simulink model "SynthFSE"  (R2019a)
settings: Solver=ode45  StartTime=0.0  StopTime=1780  RelTol=1e-3  EnableMultiTasking=on
undefined symbols (not defined in the file): j
libraries: xbsIndex_r4 x72, dspmlti4 x2, xbsCopyrightNotice_r4 x1
(part 1 of 2)
settings Model: Creator=alexc  LastModifiedBy=viswanad
settings DataIOCC: LimitDataPoints=on  SaveFormat=Array  SignalLoggingSaveFormat=ModelDataLogs  ReturnWorkspaceOutputs=off  SignalLoggingName=sigsOut
settings OptimizationCC: BlockReduction=off  BooleanDataType=off  ExpressionDepthLimit=2147483647  InitFltsAndDblsToZero=on  LifeSpan=inf
settings DebuggingCC: SaveWithParameterizedLinksMsg=none  UnderspecifiedInitializationDetection=Classic  MergeDetectMultiDrivingBlocksExec=none  SignalResolutionControl=TryResolveAllWithWarning  MultiTaskDSMMsg=warning  MultiTaskCondExecSysMsg=none  FcnCallInpInsideContextMsg=warning  StateNameClashWarn=warning  SFUnexpectedBacktrackingDiag=warning  SFNoUnconditionalDefaultTransitionDiag=warning  SFExecutionAtInitializationDiag=none  ArithmeticOperatorsInVariantConditions=warning
settings HardwareCC: ProdBitPerPointer=32  ProdBitPerSizeT=32  ProdBitPerPtrDiffT=32  ProdLargestAtomicFloat=None  ProdIntDivRoundTo=Undefined  ProdEndianess=Unspecified  ProdWordSize=32  ProdHWDeviceType=32-bit Generic  TargetUnknown=on
settings ModelReferenceCC: PropagateSignalLabelsOutOfModel=off
settings SFSimCC: SimUseLocalCustomCode=off
settings RTWCC: Description=Generic Real-Time Target  RTWUseLocalCustomCode=off
settings CodeAppCC: StateflowObjectComments=on
settings GRTTargetCC: TargetFcnLib=ansi_tfl_tmw.mat  TargetLangStandard=C89/C90 (ANSI)  GeneratePreprocessorConditionals=Disable all  CombineOutputUpdateFcns=off  GRTInterface=on
settings ConfigComp: CovMetricSettings=dw  CovHtmlReporting=on  CovSaveCumulativeToWorkspaceVar=on  CovSaveSingleToWorkspaceVar=on  CovExternalEMLEnable=off

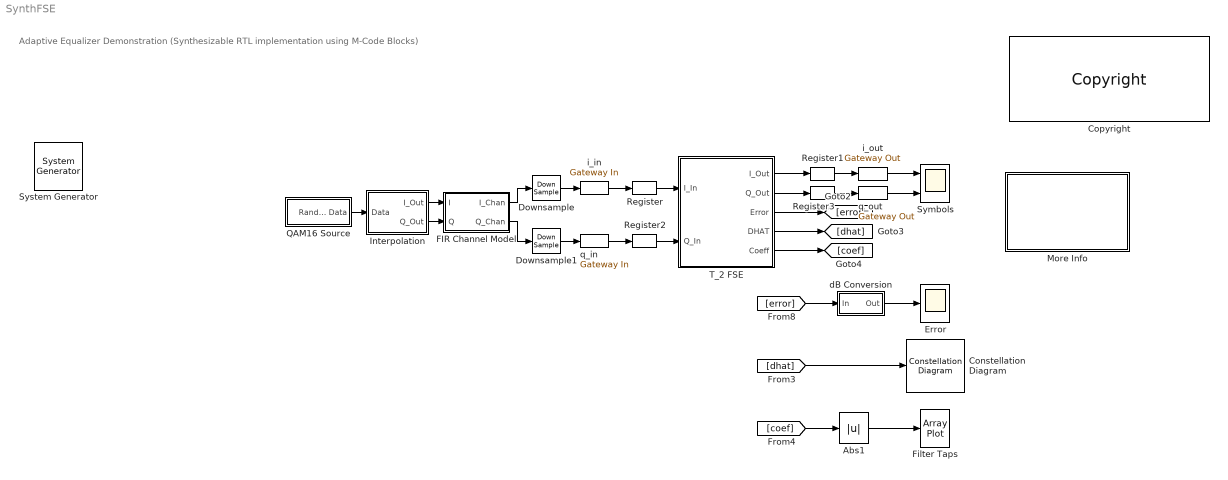
== system SynthFSE ==
  note: Adaptive Equalizer Demonstration
      | (Synthesizable RTL implementation using M-Code Blocks)
  " System Generator" : xbsIndex_r4/ System Generator  Tag=genX  xilinxfamily=kintex7  part=xc7k325t  speed=-3  package=fbg676  synthesis_tool=Vivado  clock_wrapper=Clock Enables  directory=./netlist  proj_type=Vivado  Synth_file=Vivado Synthesis Defaults  Impl_file=Vivado Implementation Defaults  testbench=off  simulink_period=1  sysclk_period=10  dcm_input_clock_period=10  incr_netlist=off  trim_vbits=Everywhere in SubSystem  dbl_ovrd=According to Block Masks  core_generation=According to Block Masks  run_coregen=off  deprecated_control=off  eval_field=0  block_type=sysgen
  Abs1 : Abs  SaturateOnIntegerOverflow=on
  Constellation Diagram : ConstellationDiagram
  Copyright : xbsCopyrightNotice_r4/Copyright  copyrighttext="Copyright (c) 2020  by  Xilinx, Inc. All rights reserved.<br><br>This file contains proprietary, confidential information of Xilinx, Inc., is distributed under license from Xilinx, Inc., and may be used, copied and/or disclosed only pursuant to the terms of a valid license agreement with Xilinx, Inc. Xilinx hereby grants you a license to use this file solely for design, simulation, implementation and creation of design files limited to Xilinx devices or technologies. Use with non-Xilinx devices or technologies is expressly prohibited and immediately terminates your license unless covered by a separate agreement.<br><br>Xilinx is providing this design, code, or information \"as-is\" solely for use in developing programs and solutions for Xilinx devices, with no obligation on the part of Xilinx to provide support. By providing this design, code, or information as one possible implementation of this feature, application or standard, Xilinx is making no representation that this implementation is free from any claims of infringement. You are responsible for obtaining any rights you may require for your implementation. Xilinx expressly disclaims any warranty whatsoever with respect to the adequacy of the implementation, including but not limited to any warranties or representations that this implementation is free from claims of infringement, implied warranties of merchantability or fitness for a particular purpose.<br><br>Xilinx products are not intended for use in life support appliances, devices, or systems. Use in such applications is expressly prohibited.<br><br>Any modifications that are made to the Source Code are done at the user's sole risk and will be unsupported.<br><br>This copyright and support notice must be retained as part of this text at all times. (c) Copyright 1995-2020 Xilinx, Inc. All rights reserved."  block_type=copyright
      settings: block_version=10.1.00
      settings: infoedit=|
      | Copyright(C) 2008 by  Xilinx, Inc. All rights reserved.<br>
      | <br>
      | This file contains proprietary, confidential information of Xilinx, Inc., is distributed under license
      | from Xilinx, Inc., and may be used, copied and/or disclosed only pursuant to the terms of a valid license
      | agreement with Xilinx, Inc. Xilinx hereby grants you a license to use this file solely for design,
      | simulation, implementation and creation of design files limited to Xilinx devices or technologies. Use
      | with non-Xilinx devices or technologies is expressly prohibited and immediately terminates your license
      | unless covered by a separate agreement.<br>
      | <br>
      | Xilinx is providing this design, code, or information "as-is" solely for use in developing programs and
      | solutions for Xilinx devices, with no obligation on the part of Xilinx to provide support. By providing
      | this design, code, or information as one possible implementation of this feature, application or standard,
      | Xilinx is making no representation that this implementation is free from any claims of infringement. You
      | are responsible for obtaining any rights you may require for your implementation. Xilinx expressly disclaims
      | any warranty whatsoever with respect to the adequacy of the implementation, including but not limited to any
      | warranties or representations that this implementation is free from claims of infringement, implied warranties
      | of merchantability or fitness for a particular purpose.<br>
      | <br>
      | Xilinx products are not intended for use in life support appliances, devices, or systems. Use in such
      | applications is expressly prohibited.<br>
      | <br>
      | Any modifications that are made to the Source Code are done at the user's sole risk and will be unsupported.<br>
      | <br>
      | This copyright and support notice must be retained as part of this text at all times.
      | (c) Copyright 1995-2008 Xilinx, Inc. All rights reserved.
  Downsample : DownSample  RateOptions=Allow multirate processing
  Downsample1 : DownSample  RateOptions=Allow multirate processing
  Error : Scope
  FIR Channel Model : Subsystem  mask{chan=[1+j*0.1 .2 j*0.2 0 0 0 0 0 0 0]}
      mask prompts: chan "Channel"
  Filter Taps : ArrayPlot
  Interpolation : Subsystem
  More Info : Subsystem
      mask Display: disp('Double click\n for\n more information.')
  QAM16 Source : Subsystem
  Register{,1..3} (4 alike) : xbsIndex_r4/Register  init=0  rst=off  en=off  dbl_ovrd=off  block_type=register
      Register settings: xl_area=[6 12 0 0 0 0 0]  block_version=VER_STRING_GOES_HERE
      Register1 settings: xl_area=[5 10 0 0 0 0 0]  block_version=VER_STRING_GOES_HERE
      Register2 settings: xl_area=[6 12 0 0 0 0 0]  block_version=VER_STRING_GOES_HERE
      Register3 settings: xl_area=[5 10 0 0 0 0 0]  block_version=VER_STRING_GOES_HERE
  Symbols : Scope  NumInputPorts=2
  T_2 FSE : Subsystem  mask{mu=.005}
  dB Conversion : Subsystem
  i_in : xbsIndex_r4/Gateway In  gui_display_data_type=Fixed-point  arith_type="Signed  (2's comp)"  n_bits=12  bin_pt=10  preci_type=Single  exp_width=8  frac_width=24  rows=1  columns=1  quantization="Round  (unbiased: +/- Inf)"  overflow=Saturate  period=2  UseAsADC=off  ADCChannel='1'  interface=None  automatic_assignment=on  address_offset=hex2dec('00')  intf_name=''  intf_description=''  default_value=0  timing_constraint=None  locs_specified=off  LOCs={}  io_standard={}  inherit_from_input=off  hdl_port=on  dbl_ovrd=off  block_type=gatewayin
      settings: infoedit="Gateway in block.  Converts inputs of type Simulink integer, double and fixed point to  Xilinx fixed point type.<P><P>Hardware notes:  In hardware these blocks become top level input ports."  xl_area=[0 0 0 0 12 0 0]  block_version=VER_STRING_GOES_HERE
  i_out : xbsIndex_r4/Gateway Out  inherit_from_input=off  hdl_port=on  rows=1  columns=1  UseAsDAC=off  DACChannel='1'  interface=None  automatic_assignment=on  address_offset=hex2dec('00')  intf_name=''  intf_description=''  timing_constraint="Data Rate;  Set 'FAST' Attribute"  locs_specified=off  LOCs={}  io_standard={}  block_type=gatewayout
      settings: infoedit="Gateway out block.  Converts Xilinx fixed point inputs into ouputs of type Simulink integer, double, or fixed point.<P><P>Hardware notes:  In hardware these blocks become top level output ports or are discarded, depending on how they are configured."  xl_area=[0 0 0 0 10 0 0]  block_version=VER_STRING_GOES_HERE
  q_in : xbsIndex_r4/Gateway In  gui_display_data_type=Fixed-point  arith_type="Signed  (2's comp)"  n_bits=12  bin_pt=10  preci_type=Single  exp_width=8  frac_width=24  rows=1  columns=1  quantization="Round  (unbiased: +/- Inf)"  overflow=Saturate  period=2  UseAsADC=off  ADCChannel='1'  interface=None  automatic_assignment=on  address_offset=hex2dec('00')  intf_name=''  intf_description=''  default_value=0  timing_constraint=None  locs_specified=off  LOCs={}  io_standard={}  inherit_from_input=off  hdl_port=on  dbl_ovrd=off  block_type=gatewayin
      settings: infoedit="Gateway in block.  Converts inputs of type Simulink integer, double and fixed point to  Xilinx fixed point type.<P><P>Hardware notes:  In hardware these blocks become top level input ports."  xl_area=[0 0 0 0 12 0 0]  block_version=VER_STRING_GOES_HERE
  q_out : xbsIndex_r4/Gateway Out  inherit_from_input=off  hdl_port=on  rows=1  columns=1  UseAsDAC=off  DACChannel='1'  interface=None  automatic_assignment=on  address_offset=hex2dec('00')  intf_name=''  intf_description=''  timing_constraint="Data Rate;  Set 'FAST' Attribute"  locs_specified=off  LOCs={}  io_standard={}  block_type=gatewayout
      settings: infoedit="Gateway out block.  Converts Xilinx fixed point inputs into ouputs of type Simulink integer, double, or fixed point.<P><P>Hardware notes:  In hardware these blocks become top level output ports or are discarded, depending on how they are configured."  xl_area=[0 0 0 0 10 0 0]  block_version=VER_STRING_GOES_HERE
  wires:
  QAM16 Source/1(" Random Data") -> Interpolation/1(Data)
  Interpolation/2(Q_Out) -> FIR Channel Model/2(Q)
  T_2 FSE/3(Error) -> [error]
  Downsample1/1 -> q_in/1
  Downsample/1 -> i_in/1
  Interpolation/1(I_Out) -> FIR Channel Model/1(I)
  T_2 FSE/2(Q_Out) -> Register3/1
  T_2 FSE/1(I_Out) -> Register1/1
  FIR Channel Model/1(I_Chan) -> Downsample/1
  FIR Channel Model/2(Q_Chan) -> Downsample1/1
  T_2 FSE/5(Coeff) -> [coef]
  i_in/1 -> Register/1
  Abs1/1 -> Filter Taps/1
  T_2 FSE/4(DHAT) -> [dhat]
  dB Conversion/1(Out) -> Error/1
  Register2/1 -> T_2 FSE/2(Q_In)
  Register1/1 -> i_out/1
  Register3/1 -> q_out/1
  q_in/1 -> Register2/1
  Register/1 -> T_2 FSE/1(I_In)
  [coef] -> Abs1/1
  [dhat] -> Constellation Diagram/1
  [error] -> dB Conversion/1(In)
  i_out/1 -> Symbols/1
  q_out/1 -> Symbols/2

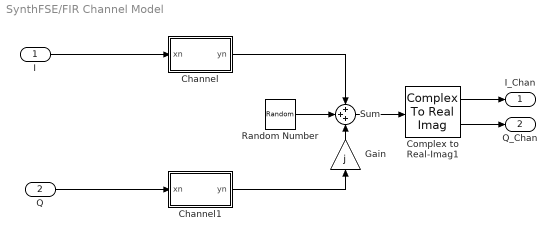
== system SynthFSE/FIR Channel Model ==
  I : Inport
  Q : Inport  Port=2
  Channel : Subsystem
  Channel1 : Subsystem
  Complex to Real-Imag1 : ComplexToRealImag
  Gain : Gain  Gain=j  SaturateOnIntegerOverflow=on  OutDataTypeStr=Inherit: Same as input  ParamDataTypeStr=Inherit: Same as input
  Random Number : RandomNumber  Variance=.01  SampleTime=100000
  Sum : Sum  Inputs=+++  SaturateOnIntegerOverflow=on  InputSameDT=on  OutDataTypeStr=Inherit: Same as first input
  I_Chan : Outport
  Q_Chan : Outport  Port=2
  wires:
  Channel1/1(yn) -> Gain/1
  Channel/1(yn) -> Sum/1
  Q/1 -> Channel1/1(xn)
  I/1 -> Channel/1(xn)
  Random Number/1 -> Sum/2
  Gain/1 -> Sum/3
  Sum/1 -> Complex to Real-Imag1/1
  Complex to Real-Imag1/2 -> Q_Chan/1
  Complex to Real-Imag1/1 -> I_Chan/1

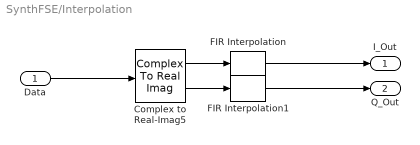
== system SynthFSE/Interpolation ==
  Data : Inport
  Complex to Real-Imag5 : ComplexToRealImag
  FIR Interpolation : dspmlti4/FIR Interpolation  FilterSource=Dialog parameters  h=sinc(-3:.25:3);  L=4  FilterObject=Hm_firinterp  framing=Allow multirate processing  outputBufInitCond=0  roundingMode=Floor  overflowMode=off  firstCoeffDataTypeStr=Inherit: Same word length as input  firstCoeffMin=[]  firstCoeffMax=[]  firstCoeffLastDataTypeStr=Inherit: Same word length as input  outputDataTypeStr=Inherit: Same as accumulator  outputMin=[]  outputMax=[]  outputLastDataTypeStr=Inherit: Same as accumulator
      settings: SourceProductName=DSP System Toolbox
  FIR Interpolation1 : dspmlti4/FIR Interpolation  FilterSource=Dialog parameters  h=sinc(-3:.25:3);  L=4  FilterObject=Hm_firinterp  framing=Allow multirate processing  outputBufInitCond=0  roundingMode=Floor  overflowMode=off  firstCoeffDataTypeStr=Inherit: Same word length as input  firstCoeffMin=[]  firstCoeffMax=[]  firstCoeffLastDataTypeStr=Inherit: Same word length as input  outputDataTypeStr=Inherit: Same as accumulator  outputMin=[]  outputMax=[]  outputLastDataTypeStr=Inherit: Same as accumulator
      settings: SourceProductName=DSP System Toolbox
  I_Out : Outport
  Q_Out : Outport  Port=2
  wires:
  Complex to Real-Imag5/2 -> FIR Interpolation1/1
  Complex to Real-Imag5/1 -> FIR Interpolation/1
  FIR Interpolation/1 -> I_Out/1
  Data/1 -> Complex to Real-Imag5/1
  FIR Interpolation1/1 -> Q_Out/1

== system SynthFSE/More Info ==
  note: This design shows a T/2 adaptive Fractionally Space Equalizer (FSE)
      | operating on a 16-QAM data source with noise and filtering introduced
      | in the channel model.  The two 4-tap FIR filters are based on an
      | SRL16E-based MAC implementation.
      |
      | The DHAT scope provides an X-Y plot of the I and Q filter outputs from
      | within the FSE.  As the simulation progresses, these symbols will
      | converge as the error is reduced.  The magnitude of the filter coefficients
      | is shown in a vector scope as well.  Increasing the simulation duration
      | will allow better visualization of the adaptive FSE effects on the filter output.
      |
      | For additional information on FSE:
      |
      | J.R. Treichler, I. Fijalkow, and C.R. Johnson, Jr.  "Fractionally Spaced
      | Equalizers"  IEEE Signal Processing Magazine, May 1996, pp. 65-81.
      |
      | Chris H. Dick, "Design and implementation of high-performance FPGA
      | signal processing datapaths for software-defined radios" VMEbus
      | Systems, August 2001.
  note: Adaptive FSE Demonstration Using a 16-QAM Source

== system SynthFSE/QAM16 Source ==
  QAM16 - I : Subsystem
  QAM16 -Q : Subsystem
  Real-Imag to Complex : RealImagToComplex
  " Random Data" : Outport
  wires:
  QAM16 - I/1(I) -> Real-Imag to Complex/1
  QAM16 -Q/1(Q) -> Real-Imag to Complex/2
  Real-Imag to Complex/1 -> " Random Data"/1

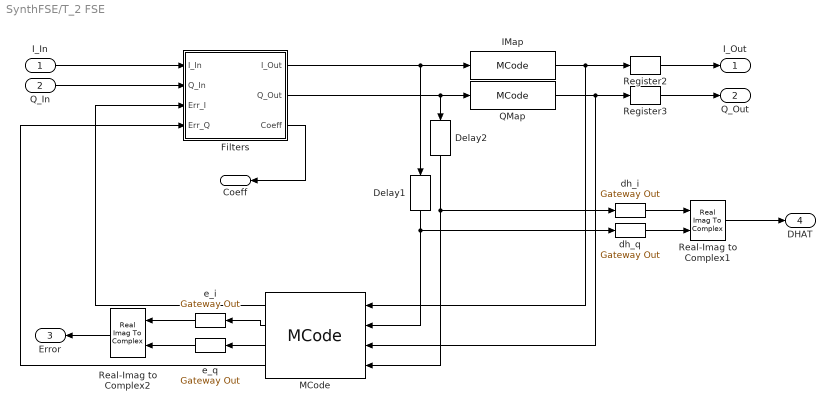
== system SynthFSE/T_2 FSE ==
  I_In : Inport
  Q_In : Inport  Port=2
  Delay1 : xbsIndex_r4/Delay  rst=off  infoeditControl=Selection of Reset will increase slice count due to use of real FFs and instead of SRLs  en=off  latency=2  reg_retiming=on  dbl_ovrd=off  block_type=delay
      settings: infoedit="Delay line having  configurable length.<P><P>Hardware notes: A delay line is a chain, each link of which is an SRL16 followed by a flip-flop. If register retiming is enabled, the delay line is a chain of flip-flops."  xl_area=[9 18 0 18 0 0 0]  block_version=VER_STRING_GOES_HERE
  Delay2 : xbsIndex_r4/Delay  rst=off  infoeditControl=Selection of Reset will increase slice count due to use of real FFs and instead of SRLs  en=off  latency=2  reg_retiming=on  dbl_ovrd=off  block_type=delay
      settings: infoedit="Delay line having  configurable length.<P><P>Hardware notes: A delay line is a chain, each link of which is an SRL16 followed by a flip-flop. If register retiming is enabled, the delay line is a chain of flip-flops."  xl_area=[9 18 0 18 0 0 0]  block_version=VER_STRING_GOES_HERE
  Filters : Subsystem
  IMap : xbsIndex_r4/MCode  mfname=QAM4map  explicit_period=off  period=1  enable_stdout=off  enable_debug=off  suppress_output=off  defparams={}  hide_port_list={}  dbl_ovrd=off  block_type=mcode
      settings: xl_area=[0, 0, 0, 0, 0, 0, 0]  block_version=8.1
  MCode : xbsIndex_r4/MCode  mfname=lmsErr  explicit_period=off  period=1  inputsTable={'boundInpExpr'=>['','','','','mu'],'inputs'=>['sym_i','filt_i','sym_q','filt_q','mu']}  outputsTable={'outputs'=>['mu_e_i','e_i','e_q','mu_e_q'],'suppressOut'=>['off','off','off','off']}  enable_stdout=off  enable_debug=off  suppress_output=1  defparams={'mu',mu}  hide_port_list={}  dbl_ovrd=off  block_type=mcode
      settings: block_version=8.2.EA1
  QMap : xbsIndex_r4/MCode  mfname=QAM4map  explicit_period=off  period=1  enable_stdout=off  enable_debug=off  suppress_output=off  defparams={}  hide_port_list={}  dbl_ovrd=off  block_type=mcode
      settings: xl_area=[0, 0, 0, 0, 0, 0, 0]  block_version=8.1
  Real-Imag to Complex1 : RealImagToComplex
  Real-Imag to Complex2 : RealImagToComplex
  Register2 : xbsIndex_r4/Register  init=0  rst=off  en=off  dbl_ovrd=off  block_type=register
      settings: xl_area=[5 10 0 0 0 0 0]  block_version=VER_STRING_GOES_HERE
  Register3 : xbsIndex_r4/Register  init=0  rst=off  en=off  dbl_ovrd=off  block_type=register
      settings: xl_area=[5 10 0 0 0 0 0]  block_version=VER_STRING_GOES_HERE
  dh_i : xbsIndex_r4/Gateway Out  inherit_from_input=off  hdl_port=off  rows=1  columns=1  UseAsDAC=off  DACChannel='1'  interface=None  automatic_assignment=on  address_offset=hex2dec('00')  intf_name=''  intf_description=''  timing_constraint=None  locs_specified=off  LOCs={}  io_standard={}  block_type=gatewayout
      settings: infoedit="Gateway out block.  Converts Xilinx fixed point inputs into ouputs of type Simulink integer, double, or fixed point.<P><P>Hardware notes:  In hardware these blocks become top level output ports or are discarded, depending on how they are configured."  xl_area=[0 0 0 0 0 0 0]  block_version=VER_STRING_GOES_HERE
  dh_q : xbsIndex_r4/Gateway Out  inherit_from_input=off  hdl_port=off  rows=1  columns=1  UseAsDAC=off  DACChannel='1'  interface=None  automatic_assignment=on  address_offset=hex2dec('00')  intf_name=''  intf_description=''  timing_constraint=None  locs_specified=off  LOCs={}  io_standard={}  block_type=gatewayout
      settings: infoedit="Gateway out block.  Converts Xilinx fixed point inputs into ouputs of type Simulink integer, double, or fixed point.<P><P>Hardware notes:  In hardware these blocks become top level output ports or are discarded, depending on how they are configured."  xl_area=[0 0 0 0 0 0 0]  block_version=VER_STRING_GOES_HERE
  e_i : xbsIndex_r4/Gateway Out  inherit_from_input=off  hdl_port=off  rows=1  columns=1  UseAsDAC=off  DACChannel='1'  interface=None  automatic_assignment=on  address_offset=hex2dec('00')  intf_name=''  intf_description=''  timing_constraint=None  locs_specified=off  LOCs={}  io_standard={}  block_type=gatewayout
      settings: infoedit="Gateway out block.  Converts Xilinx fixed point inputs into ouputs of type Simulink integer, double, or fixed point.<P><P>Hardware notes:  In hardware these blocks become top level output ports or are discarded, depending on how they are configured."  xl_area=[0 0 0 0 0 0 0]  block_version=VER_STRING_GOES_HERE
  e_q : xbsIndex_r4/Gateway Out  inherit_from_input=off  hdl_port=off  rows=1  columns=1  UseAsDAC=off  DACChannel='1'  interface=None  automatic_assignment=on  address_offset=hex2dec('00')  intf_name=''  intf_description=''  timing_constraint=None  locs_specified=off  LOCs={}  io_standard={}  block_type=gatewayout
      settings: infoedit="Gateway out block.  Converts Xilinx fixed point inputs into ouputs of type Simulink integer, double, or fixed point.<P><P>Hardware notes:  In hardware these blocks become top level output ports or are discarded, depending on how they are configured."  xl_area=[0 0 0 0 0 0 0]  block_version=VER_STRING_GOES_HERE
  I_Out : Outport
  Q_Out : Outport  Port=2
  Error : Outport  Port=3
  DHAT : Outport  Port=4
  Coeff : Outport  Port=5
  wires:
  Q_In/1 -> Filters/2(Q_In)
  Filters/1(I_Out) -> Delay1/1, IMap/1
  QMap/1 -> Register3/1, MCode/3
  IMap/1 -> Register2/1, MCode/1
  Filters/2(Q_Out) -> Delay2/1, QMap/1
  I_In/1 -> Filters/1(I_In)
  Delay1/1 -> dh_q/1, MCode/2
  Delay2/1 -> dh_i/1, MCode/4
  Real-Imag to Complex1/1 -> DHAT/1
  dh_i/1 -> Real-Imag to Complex1/1
  dh_q/1 -> Real-Imag to Complex1/2
  Filters/3(Coeff) -> Coeff/1
  Register2/1 -> I_Out/1
  Register3/1 -> Q_Out/1
  e_i/1 -> Real-Imag to Complex2/1
  e_q/1 -> Real-Imag to Complex2/2
  MCode/2 -> e_i/1
  MCode/3 -> e_q/1
  Real-Imag to Complex2/1 -> Error/1
  MCode/1 -> Filters/3(Err_I)
  MCode/4 -> Filters/4(Err_Q)

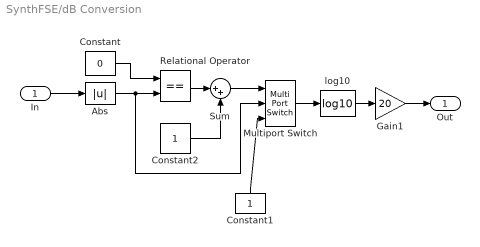
== system SynthFSE/dB Conversion ==
  In : Inport
  Abs : Abs  SaturateOnIntegerOverflow=on
  Constant : Constant  Value=0
  Constant1 : Constant
  Constant2 : Constant
  Gain1 : Gain  Gain=20  SaturateOnIntegerOverflow=on  OutDataTypeStr=Inherit: Same as input  ParamDataTypeStr=Inherit: Same as input
  Multiport Switch : MultiPortSwitch  Inputs=2  SaturateOnIntegerOverflow=on  InputSameDT=on
  Relational Operator : RelationalOperator  Operator===  RndMeth=Nearest  InputSameDT=on
  Sum : Sum  Inputs=|++  SaturateOnIntegerOverflow=on  InputSameDT=on  OutDataTypeStr=Inherit: Same as first input
  log10 : Math  Operator=log10  SaturateOnIntegerOverflow=on
  Out : Outport
  wires:
  Multiport Switch/1 -> log10/1
  Constant1/1 -> Multiport Switch/3
  Constant/1 -> Relational Operator/1
  Abs/1 -> Multiport Switch/2, Relational Operator/2
  Constant2/1 -> Sum/2
  Sum/1 -> Multiport Switch/1
  Relational Operator/1 -> Sum/1
  Gain1/1 -> Out/1
  In/1 -> Abs/1
  log10/1 -> Gain1/1

== system SynthFSE/FIR Channel Model/Channel ==
  xn : Inport
  Chan Re : Subsystem
  yn : Outport
  wires:
  xn/1 -> Chan Re/1(Input)
  Chan Re/1(Output) -> yn/1

== system SynthFSE/FIR Channel Model/Channel1 ==
  xn : Inport
  Chan Re : Subsystem
  yn : Outport
  wires:
  xn/1 -> Chan Re/1(Input)
  Chan Re/1(Output) -> yn/1

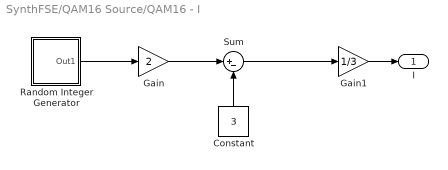
== system SynthFSE/QAM16 Source/QAM16 - I ==
  Constant : Constant  Value=3
  Gain : Gain  Gain=2  SaturateOnIntegerOverflow=on  OutDataTypeStr=Inherit: Same as input  ParamDataTypeStr=Inherit: Same as input
  Gain1 : Gain  Gain=1/3  SaturateOnIntegerOverflow=on  OutDataTypeStr=Inherit: Same as input  ParamDataTypeStr=Inherit: Same as input
  Random Integer Generator : Subsystem  mask{M=4, seed=1, Ts=4}
      mask prompts: M "M-ary Number"; seed "Initial seed"; Ts "Sample Time"
  Sum : Sum  Inputs=|+-  SaturateOnIntegerOverflow=on  InputSameDT=on  OutDataTypeStr=Inherit: Same as first input
  I : Outport
  wires:
  Random Integer Generator/1(Out1) -> Gain/1
  Gain/1 -> Sum/1
  Constant/1 -> Sum/2
  Sum/1 -> Gain1/1
  Gain1/1 -> I/1

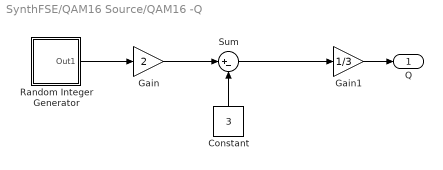
== system SynthFSE/QAM16 Source/QAM16 -Q ==
  Constant : Constant  Value=3
  Gain : Gain  Gain=2  SaturateOnIntegerOverflow=on  OutDataTypeStr=Inherit: Same as input  ParamDataTypeStr=Inherit: Same as input
  Gain1 : Gain  Gain=1/3  SaturateOnIntegerOverflow=on  OutDataTypeStr=Inherit: Same as input  ParamDataTypeStr=Inherit: Same as input
  Random Integer Generator : Subsystem  mask{M=4, seed=4, Ts=4}
      mask prompts: M "M-ary Number"; seed "Initial seed"; Ts "Sample Time"
  Sum : Sum  Inputs=|+-  SaturateOnIntegerOverflow=on  InputSameDT=on  OutDataTypeStr=Inherit: Same as first input
  Q : Outport
  wires:
  Random Integer Generator/1(Out1) -> Gain/1
  Gain/1 -> Sum/1
  Constant/1 -> Sum/2
  Sum/1 -> Gain1/1
  Gain1/1 -> Q/1

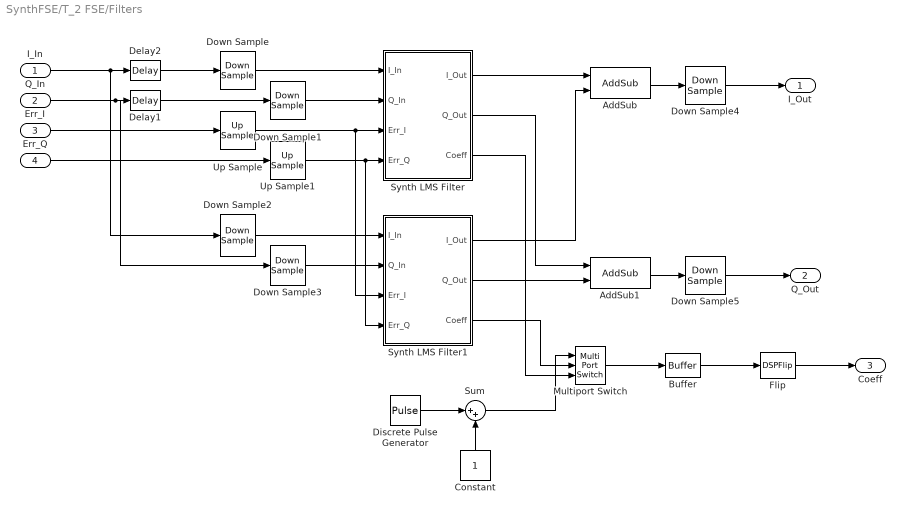
== system SynthFSE/T_2 FSE/Filters ==
  I_In : Inport
  Q_In : Inport  Port=2
  Err_I : Inport  Port=3
  Err_Q : Inport  Port=4
  AddSub : xbsIndex_r4/AddSub  mode=Addition  use_carryin=off  use_carryout=off  en=off  latency=0  precision=User Defined  arith_type="Signed  (2's comp)"  n_bits=18  bin_pt=10  quantization=Truncate  overflow=Wrap  use_behavioral_HDL=on  hw_selection=Fabric  pipelined=off  use_rpm=on  dbl_ovrd=off  block_type=addsub
      settings: block_version=VER_STRING_GOES_HERE
  AddSub1 : xbsIndex_r4/AddSub  mode=Addition  use_carryin=off  use_carryout=off  en=off  latency=0  precision=User Defined  arith_type="Signed  (2's comp)"  n_bits=18  bin_pt=10  quantization=Truncate  overflow=Wrap  use_behavioral_HDL=on  hw_selection=Fabric  pipelined=off  use_rpm=on  dbl_ovrd=off  block_type=addsub
      settings: block_version=VER_STRING_GOES_HERE
  Buffer : Buffer  N=8
  Constant : Constant
  Delay1 : xbsIndex_r4/Delay  rst=off  infoeditControl=Selection of Reset will increase slice count due to use of real FFs and instead of SRLs  en=off  latency=1  reg_retiming=on  dbl_ovrd=off  block_type=delay
      settings: infoedit="Delay line having  configurable length.<P><P>Hardware notes: A delay line is a chain, each link of which is an SRL16 followed by a flip-flop. If register retiming is enabled, the delay line is a chain of flip-flops."  xl_area=[6 12 0 0 0 0 0]  block_version=VER_STRING_GOES_HERE
  Delay2 : xbsIndex_r4/Delay  rst=off  infoeditControl=Selection of Reset will increase slice count due to use of real FFs and instead of SRLs  en=off  latency=1  reg_retiming=on  dbl_ovrd=off  block_type=delay
      settings: infoedit="Delay line having  configurable length.<P><P>Hardware notes: A delay line is a chain, each link of which is an SRL16 followed by a flip-flop. If register retiming is enabled, the delay line is a chain of flip-flops."  xl_area=[6 12 0 0 0 0 0]  block_version=VER_STRING_GOES_HERE
  Discrete Pulse Generator : DiscretePulseGenerator  SampleTime=.5
  Down Sample : xbsIndex_r4/Down Sample  sample_ratio=2  sample_phase="Last Value of Frame  (most efficient)"  en=off  rst=off  latency=1  dbl_ovrd=off  block_type=dsamp
      settings: xl_area=[6 12 0 0 0 0 0]  block_version=VER_STRING_GOES_HERE
  Down Sample1 : xbsIndex_r4/Down Sample  sample_ratio=2  sample_phase="Last Value of Frame  (most efficient)"  en=off  rst=off  latency=1  dbl_ovrd=off  block_type=dsamp
      settings: xl_area=[6 12 0 0 0 0 0]  block_version=VER_STRING_GOES_HERE
  Down Sample2 : xbsIndex_r4/Down Sample  sample_ratio=2  sample_phase="Last Value of Frame  (most efficient)"  en=off  rst=off  latency=2  dbl_ovrd=off  block_type=dsamp
      settings: xl_area=[6 12 0 12 0 0 0]  block_version=VER_STRING_GOES_HERE
  Down Sample3 : xbsIndex_r4/Down Sample  sample_ratio=2  sample_phase="Last Value of Frame  (most efficient)"  en=off  rst=off  latency=2  dbl_ovrd=off  block_type=dsamp
      settings: xl_area=[6 12 0 12 0 0 0]  block_version=VER_STRING_GOES_HERE
  Down Sample4 : xbsIndex_r4/Down Sample  sample_ratio=4  sample_phase="Last Value of Frame  (most efficient)"  en=off  rst=off  latency=1  dbl_ovrd=off  block_type=dsamp
      settings: xl_area=[9 18 0 0 0 0 0]  block_version=VER_STRING_GOES_HERE
  Down Sample5 : xbsIndex_r4/Down Sample  sample_ratio=4  sample_phase="Last Value of Frame  (most efficient)"  en=off  rst=off  latency=1  dbl_ovrd=off  block_type=dsamp
      settings: xl_area=[9 18 0 0 0 0 0]  block_version=VER_STRING_GOES_HERE
  Flip : DSPFlip
  Multiport Switch : MultiPortSwitch  Inputs=2  SaturateOnIntegerOverflow=on  InputSameDT=on
  Sum : Sum  Inputs=|++  SaturateOnIntegerOverflow=on  InputSameDT=on  OutDataTypeStr=Inherit: Same as first input
  Synth LMS Filter : Subsystem  mask{init_i=[0 0 0 0], init_q=[0 0 0 0]}
      mask prompts: init_i "Init I"; init_q "Init Q"
  Synth LMS Filter1 : Subsystem  mask{init_i=[0 1 0 0], init_q=[0 0 0 0]}
      mask prompts: init_i "Init I"; init_q "Init Q"
  Up Sample : xbsIndex_r4/Up Sample  sample_ratio=4  copy_samples=on  en=off  latency=0  dbl_ovrd=off  block_type=usamp
      settings: infoedit="Up samples input data.  Inserted values  can be zeros or copies of the most recent input sample.<P><P>Hardware notes: No hardware is needed if inserted values are copies of the input sample; otherwise, a mux and single bit flip-flop are used."  xl_area=[0 0 0 0 0 0 0]  block_version=VER_STRING_GOES_HERE
  Up Sample1 : xbsIndex_r4/Up Sample  sample_ratio=4  copy_samples=on  en=off  latency=0  dbl_ovrd=off  block_type=usamp
      settings: infoedit="Up samples input data.  Inserted values  can be zeros or copies of the most recent input sample.<P><P>Hardware notes: No hardware is needed if inserted values are copies of the input sample; otherwise, a mux and single bit flip-flop are used."  xl_area=[0 0 0 0 0 0 0]  block_version=VER_STRING_GOES_HERE
  I_Out : Outport
  Q_Out : Outport  Port=2
  Coeff : Outport  Port=3
  wires:
  Down Sample3/1 -> Synth LMS Filter1/2(Q_In)
  Down Sample1/1 -> Synth LMS Filter/2(Q_In)
  Down Sample/1 -> Synth LMS Filter/1(I_In)
  AddSub/1 -> Down Sample4/1
  Synth LMS Filter/2(Q_Out) -> AddSub1/1
  Synth LMS Filter1/1(I_Out) -> AddSub/2
  Synth LMS Filter1/2(Q_Out) -> AddSub1/2
  AddSub1/1 -> Down Sample5/1
  Multiport Switch/1 -> Buffer/1
  Constant/1 -> Sum/2
  Discrete Pulse Generator/1 -> Sum/1
  Sum/1 -> Multiport Switch/1
  Synth LMS Filter/3(Coeff) -> Multiport Switch/3
  Synth LMS Filter1/3(Coeff) -> Multiport Switch/2
  Buffer/1 -> Flip/1
  Flip/1 -> Coeff/1
  Down Sample4/1 -> I_Out/1
  Down Sample5/1 -> Q_Out/1
  Delay2/1 -> Down Sample/1
  Delay1/1 -> Down Sample1/1
  Down Sample2/1 -> Synth LMS Filter1/1(I_In)
  Err_Q/1 -> Up Sample1/1
  Err_I/1 -> Up Sample/1
  Q_In/1 -> Delay1/1, Down Sample3/1
  I_In/1 -> Delay2/1, Down Sample2/1
  Synth LMS Filter/1(I_Out) -> AddSub/1
  Up Sample/1 -> Synth LMS Filter/3(Err_I), Synth LMS Filter1/3(Err_I)
  Up Sample1/1 -> Synth LMS Filter/4(Err_Q), Synth LMS Filter1/4(Err_Q)

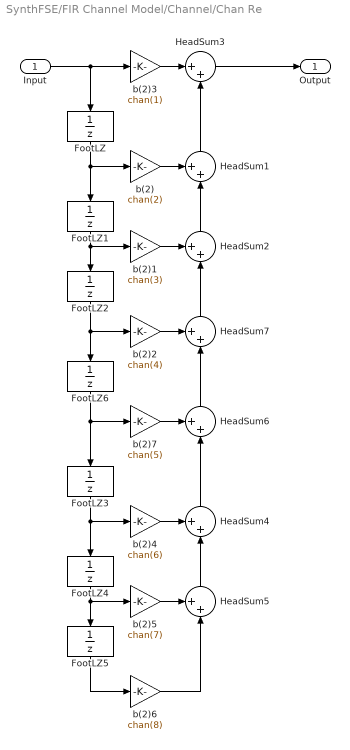
== system SynthFSE/FIR Channel Model/Channel/Chan Re ==
  Input : Inport
  FootLZ : UnitDelay  HasFrameUpgradeWarning=on
  FootLZ{1..2,4..6} (5 alike) : UnitDelay  SampleTime=-1  HasFrameUpgradeWarning=on
  FootLZ3 : UnitDelay  HasFrameUpgradeWarning=on
  HeadSum{1..2,4..7} (6 alike) : Sum  Inputs=++|  SaturateOnIntegerOverflow=on  InputSameDT=on  OutDataTypeStr=Inherit: Same as first input
  HeadSum3 : Sum  Inputs=|++  SaturateOnIntegerOverflow=on  InputSameDT=on  OutDataTypeStr=Inherit: Same as first input
  b(2) : Gain  Gain=chan(2)  SaturateOnIntegerOverflow=on  OutDataTypeStr=Inherit: Same as input  ParamDataTypeStr=Inherit: Same as input
  b(2)1 : Gain  Gain=chan(3)  SaturateOnIntegerOverflow=on  OutDataTypeStr=Inherit: Same as input  ParamDataTypeStr=Inherit: Same as input
  b(2)2 : Gain  Gain=chan(4)  SaturateOnIntegerOverflow=on  OutDataTypeStr=Inherit: Same as input  ParamDataTypeStr=Inherit: Same as input
  b(2)3 : Gain  Gain=chan(1)  SaturateOnIntegerOverflow=on  OutDataTypeStr=Inherit: Same as input  ParamDataTypeStr=Inherit: Same as input
  b(2)4 : Gain  Gain=chan(6)  SaturateOnIntegerOverflow=on  OutDataTypeStr=Inherit: Same as input  ParamDataTypeStr=Inherit: Same as input
  b(2)5 : Gain  Gain=chan(7)  SaturateOnIntegerOverflow=on  OutDataTypeStr=Inherit: Same as input  ParamDataTypeStr=Inherit: Same as input
  b(2)6 : Gain  Gain=chan(8)  SaturateOnIntegerOverflow=on  OutDataTypeStr=Inherit: Same as input  ParamDataTypeStr=Inherit: Same as input
  b(2)7 : Gain  Gain=chan(5)  SaturateOnIntegerOverflow=on  OutDataTypeStr=Inherit: Same as input  ParamDataTypeStr=Inherit: Same as input
  Output : Outport
  wires:
  HeadSum6/1 -> HeadSum7/2
  HeadSum4/1 -> HeadSum6/2
  HeadSum7/1 -> HeadSum2/2
  b(2)2/1 -> HeadSum7/1
  FootLZ6/1 -> FootLZ3/1, b(2)7/1
  FootLZ3/1 -> b(2)4/1, FootLZ4/1
  FootLZ4/1 -> FootLZ5/1, b(2)5/1
  FootLZ5/1 -> b(2)6/1
  b(2)4/1 -> HeadSum4/1
  b(2)5/1 -> HeadSum5/1
  HeadSum5/1 -> HeadSum4/2
  b(2)6/1 -> HeadSum5/2
  b(2)7/1 -> HeadSum6/1
  FootLZ2/1 -> FootLZ6/1, b(2)2/1
  FootLZ/1 -> b(2)/1, FootLZ1/1
  FootLZ1/1 -> FootLZ2/1, b(2)1/1
  b(2)/1 -> HeadSum1/1
  b(2)1/1 -> HeadSum2/1
  HeadSum2/1 -> HeadSum1/2
  Input/1 -> FootLZ/1, b(2)3/1
  b(2)3/1 -> HeadSum3/1
  HeadSum1/1 -> HeadSum3/2
  HeadSum3/1 -> Output/1

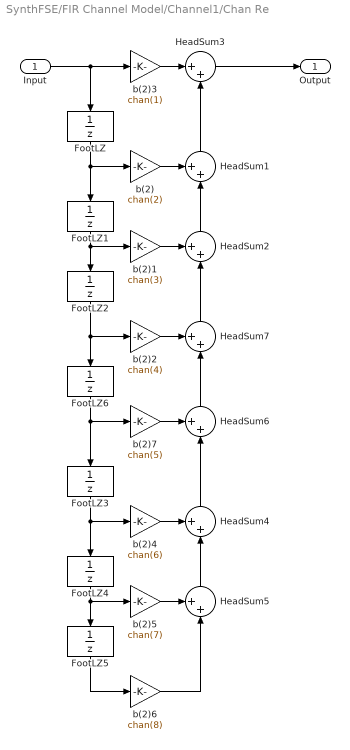
== system SynthFSE/FIR Channel Model/Channel1/Chan Re ==
  Input : Inport
  FootLZ : UnitDelay  HasFrameUpgradeWarning=on
  FootLZ{1..2,4..6} (5 alike) : UnitDelay  SampleTime=-1  HasFrameUpgradeWarning=on
  FootLZ3 : UnitDelay  HasFrameUpgradeWarning=on
  HeadSum{1..2,4..7} (6 alike) : Sum  Inputs=++|  SaturateOnIntegerOverflow=on  InputSameDT=on  OutDataTypeStr=Inherit: Same as first input
  HeadSum3 : Sum  Inputs=|++  SaturateOnIntegerOverflow=on  InputSameDT=on  OutDataTypeStr=Inherit: Same as first input
  b(2) : Gain  Gain=chan(2)  SaturateOnIntegerOverflow=on  OutDataTypeStr=Inherit: Same as input  ParamDataTypeStr=Inherit: Same as input
  b(2)1 : Gain  Gain=chan(3)  SaturateOnIntegerOverflow=on  OutDataTypeStr=Inherit: Same as input  ParamDataTypeStr=Inherit: Same as input
  b(2)2 : Gain  Gain=chan(4)  SaturateOnIntegerOverflow=on  OutDataTypeStr=Inherit: Same as input  ParamDataTypeStr=Inherit: Same as input
  b(2)3 : Gain  Gain=chan(1)  SaturateOnIntegerOverflow=on  OutDataTypeStr=Inherit: Same as input  ParamDataTypeStr=Inherit: Same as input
  b(2)4 : Gain  Gain=chan(6)  SaturateOnIntegerOverflow=on  OutDataTypeStr=Inherit: Same as input  ParamDataTypeStr=Inherit: Same as input
  b(2)5 : Gain  Gain=chan(7)  SaturateOnIntegerOverflow=on  OutDataTypeStr=Inherit: Same as input  ParamDataTypeStr=Inherit: Same as input
  b(2)6 : Gain  Gain=chan(8)  SaturateOnIntegerOverflow=on  OutDataTypeStr=Inherit: Same as input  ParamDataTypeStr=Inherit: Same as input
  b(2)7 : Gain  Gain=chan(5)  SaturateOnIntegerOverflow=on  OutDataTypeStr=Inherit: Same as input  ParamDataTypeStr=Inherit: Same as input
  Output : Outport
  wires:
  b(2)2/1 -> HeadSum7/1
  HeadSum7/1 -> HeadSum2/2
  HeadSum6/1 -> HeadSum7/2
  FootLZ6/1 -> b(2)7/1, FootLZ3/1
  FootLZ2/1 -> FootLZ6/1, b(2)2/1
  FootLZ3/1 -> b(2)4/1, FootLZ4/1
  FootLZ4/1 -> FootLZ5/1, b(2)5/1
  FootLZ5/1 -> b(2)6/1
  b(2)4/1 -> HeadSum4/1
  b(2)5/1 -> HeadSum5/1
  HeadSum5/1 -> HeadSum4/2
  b(2)6/1 -> HeadSum5/2
  b(2)7/1 -> HeadSum6/1
  HeadSum4/1 -> HeadSum6/2
  FootLZ/1 -> b(2)/1, FootLZ1/1
  FootLZ1/1 -> FootLZ2/1, b(2)1/1
  b(2)/1 -> HeadSum1/1
  b(2)1/1 -> HeadSum2/1
  HeadSum2/1 -> HeadSum1/2
  Input/1 -> FootLZ/1, b(2)3/1
  b(2)3/1 -> HeadSum3/1
  HeadSum1/1 -> HeadSum3/2
  HeadSum3/1 -> Output/1

== system SynthFSE/QAM16 Source/QAM16 - I/Random Integer Generator ==
  Rounding Function : Rounding  Operator=round
  Uniform Random Number : UniformRandomNumber  Minimum=-0.49  Maximum=M-1 + 0.49  Seed=seed  SampleTime=Ts
  Out1 : Outport
  wires:
  Rounding Function/1 -> Out1/1
  Uniform Random Number/1 -> Rounding Function/1

== system SynthFSE/QAM16 Source/QAM16 -Q/Random Integer Generator ==
  Rounding Function : Rounding  Operator=round
  Uniform Random Number : UniformRandomNumber  Minimum=-0.49  Maximum=M-1 + 0.49  Seed=seed  SampleTime=Ts
  Out1 : Outport
  wires:
  Rounding Function/1 -> Out1/1
  Uniform Random Number/1 -> Rounding Function/1

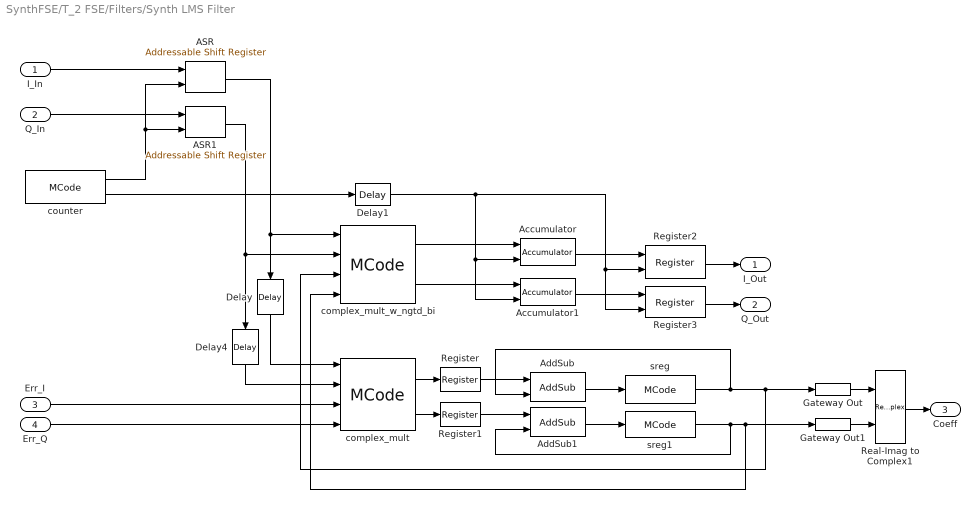
== system SynthFSE/T_2 FSE/Filters/Synth LMS Filter ==
  I_In : Inport
  Q_In : Inport  Port=2
  Err_I : Inport  Port=3
  Err_Q : Inport  Port=4
  ASR : xbsIndex_r4/Addressable Shift Register  infer_latency=off  depth=4  initVector=[0]  en=off  use_behavioral_HDL=on  Optimization=Resource  use_rpm=on  dbl_ovrd=off  block_type=addrsr
      settings: infoedit="Delay of configurable length.  Any element in the delay line can be addressed and driven onto the output port.<P><P>Hardware notes: Implemented using SRL16s.  If a Virtex-II device is used, multiple SRLC16s are cascaded together."  block_version=VER_STRING_GOES_HERE
  ASR1 : xbsIndex_r4/Addressable Shift Register  infer_latency=off  depth=4  initVector=[0]  en=off  use_behavioral_HDL=on  Optimization=Resource  use_rpm=on  dbl_ovrd=off  block_type=addrsr
      settings: infoedit="Delay of configurable length.  Any element in the delay line can be addressed and driven onto the output port.<P><P>Hardware notes: Implemented using SRL16s.  If a Virtex-II device is used, multiple SRLC16s are cascaded together."  block_version=VER_STRING_GOES_HERE
  Accumulator : xbsIndex_r4/Accumulator  operation=Add  n_bits=36  overflow=Wrap  scale=1  rst=on  hasbypass=off  infoeditControl=reset for floating point data type must be asserted for a minimum of 2 cycles  en=off  latency=1  msb_inp=100  msb=100  lsb=-100  use_behavioral_HDL=on  implementation=Fabric  dbl_ovrd=off  block_type=accum
      settings: block_version=VER_STRING_GOES_HERE
  Accumulator1 : xbsIndex_r4/Accumulator  operation=Add  n_bits=36  overflow=Wrap  scale=1  rst=on  hasbypass=off  infoeditControl=reset for floating point data type must be asserted for a minimum of 2 cycles  en=off  latency=1  msb_inp=100  msb=100  lsb=-100  use_behavioral_HDL=on  implementation=Fabric  dbl_ovrd=off  block_type=accum
      settings: block_version=VER_STRING_GOES_HERE
  AddSub : xbsIndex_r4/AddSub  mode=Addition  use_carryin=off  use_carryout=off  en=off  latency=0  precision=User Defined  arith_type="Signed  (2's comp)"  n_bits=18  bin_pt=10  quantization="Round  (unbiased: +/- Inf)"  overflow=Saturate  use_behavioral_HDL=on  hw_selection=Fabric  pipelined=off  use_rpm=on  dbl_ovrd=off  block_type=addsub
      settings: block_version=VER_STRING_GOES_HERE
  AddSub1 : xbsIndex_r4/AddSub  mode=Addition  use_carryin=off  use_carryout=off  en=off  latency=0  precision=User Defined  arith_type="Signed  (2's comp)"  n_bits=18  bin_pt=10  quantization="Round  (unbiased: +/- Inf)"  overflow=Saturate  use_behavioral_HDL=on  hw_selection=Fabric  pipelined=off  use_rpm=on  dbl_ovrd=off  block_type=addsub
      settings: block_version=VER_STRING_GOES_HERE
  Delay : xbsIndex_r4/Delay  rst=off  infoeditControl=Selection of Reset will increase slice count due to use of real FFs and instead of SRLs  en=off  latency=27  reg_retiming=off  dbl_ovrd=off  block_type=delay
      settings: infoedit="Delay line having  configurable length.<P><P>Hardware notes: A delay line is a chain, each link of which is an SRL16 followed by a flip-flop. If register retiming is enabled, the delay line is a chain of flip-flops."  xl_area=[12 24 0 24 0 0 0]  block_version=VER_STRING_GOES_HERE
  Delay1 : xbsIndex_r4/Delay  rst=off  infoeditControl=Selection of Reset will increase slice count due to use of real FFs and instead of SRLs  en=off  latency=3  reg_retiming=on  dbl_ovrd=off  block_type=delay
      settings: infoedit="Delay line having  configurable length.<P><P>Hardware notes: A delay line is a chain, each link of which is an SRL16 followed by a flip-flop. If register retiming is enabled, the delay line is a chain of flip-flops."  xl_area=[1 1 0 1 0 0 0]  block_version=VER_STRING_GOES_HERE
  Delay4 : xbsIndex_r4/Delay  rst=off  infoeditControl=Selection of Reset will increase slice count due to use of real FFs and instead of SRLs  en=off  latency=27  reg_retiming=off  dbl_ovrd=off  block_type=delay
      settings: infoedit="Delay line having  configurable length.<P><P>Hardware notes: A delay line is a chain, each link of which is an SRL16 followed by a flip-flop. If register retiming is enabled, the delay line is a chain of flip-flops."  xl_area=[12 24 0 24 0 0 0]  block_version=VER_STRING_GOES_HERE
  Gateway Out : xbsIndex_r4/Gateway Out  inherit_from_input=off  hdl_port=off  rows=1  columns=1  UseAsDAC=off  DACChannel='1'  interface=None  automatic_assignment=on  address_offset=hex2dec('00')  intf_name=''  intf_description=''  timing_constraint=None  locs_specified=off  LOCs={}  io_standard={}  block_type=gatewayout
      settings: infoedit="Gateway out block.  Converts Xilinx fixed point inputs into ouputs of type Simulink integer, double, or fixed point.<P><P>Hardware notes:  In hardware these blocks become top level output ports or are discarded, depending on how they are configured."  xl_area=[0 0 0 0 0 0 0]  block_version=VER_STRING_GOES_HERE
  Gateway Out1 : xbsIndex_r4/Gateway Out  inherit_from_input=off  hdl_port=off  rows=1  columns=1  UseAsDAC=off  DACChannel='1'  interface=None  automatic_assignment=on  address_offset=hex2dec('00')  intf_name=''  intf_description=''  timing_constraint=None  locs_specified=off  LOCs={}  io_standard={}  block_type=gatewayout
      settings: infoedit="Gateway out block.  Converts Xilinx fixed point inputs into ouputs of type Simulink integer, double, or fixed point.<P><P>Hardware notes:  In hardware these blocks become top level output ports or are discarded, depending on how they are configured."  xl_area=[0 0 0 0 0 0 0]  block_version=VER_STRING_GOES_HERE
  Real-Imag to Complex1 : RealImagToComplex
  Register : xbsIndex_r4/Register  init=0  rst=off  en=off  dbl_ovrd=off  block_type=register
      settings: xl_area=[18 36 0 0 0 0 0]  block_version=VER_STRING_GOES_HERE
  Register1 : xbsIndex_r4/Register  init=0  rst=off  en=off  dbl_ovrd=off  block_type=register
      settings: xl_area=[18 36 0 0 0 0 0]  block_version=VER_STRING_GOES_HERE
  Register2 : xbsIndex_r4/Register  init=0  rst=off  en=on  dbl_ovrd=off  block_type=register
      settings: xl_area=[18 36 0 0 0 0 0]  block_version=VER_STRING_GOES_HERE
  Register3 : xbsIndex_r4/Register  init=0  rst=off  en=on  dbl_ovrd=off  block_type=register
      settings: xl_area=[18 36 0 0 0 0 0]  block_version=VER_STRING_GOES_HERE
  complex_mult : xbsIndex_r4/MCode  mfname=complex_mult  explicit_period=off  period=1  enable_stdout=off  enable_debug=off  suppress_output=off  defparams={'negate_bi', 0}  hide_port_list={}  dbl_ovrd=off  block_type=mcode
      settings: xl_area=[0, 0, 0, 0, 0, 0, 0]  block_version=8.1
  complex_mult_w_ngtd_bi : xbsIndex_r4/MCode  mfname=complex_mult  explicit_period=off  period=1  enable_stdout=off  enable_debug=off  suppress_output=off  defparams={'negate_bi', 1}  hide_port_list={}  dbl_ovrd=off  block_type=mcode
      settings: xl_area=[0, 0, 0, 0, 0, 0, 0]  block_version=8.1
  counter : xbsIndex_r4/MCode  mfname=fir_fsm  explicit_period=on  period=1  enable_stdout=off  enable_debug=off  suppress_output=off  defparams={'reset', false,'init', 3}  hide_port_list={}  dbl_ovrd=off  block_type=mcode
      settings: xl_area=[0, 0, 0, 0, 0, 0, 0]  block_version=8.1
  sreg : xbsIndex_r4/MCode  mfname=sreg  explicit_period=off  period=1  enable_stdout=off  enable_debug=off  suppress_output=off  defparams={'len',4,'init',init_i}  hide_port_list={}  dbl_ovrd=off  block_type=mcode
      settings: xl_area=[0, 0, 0, 0, 0, 0, 0]  block_version=8.1
  sreg1 : xbsIndex_r4/MCode  mfname=sreg  explicit_period=off  period=1  enable_stdout=off  enable_debug=off  suppress_output=off  defparams={'len',4,'init',init_q}  hide_port_list={}  dbl_ovrd=off  block_type=mcode
      settings: xl_area=[0, 0, 0, 0, 0, 0, 0]  block_version=8.1
  I_Out : Outport
  Q_Out : Outport  Port=2
  Coeff : Outport  Port=3
  wires:
  Q_In/1 -> ASR1/1
  I_In/1 -> ASR/1
  ASR1/1 -> complex_mult_w_ngtd_bi/2, Delay4/1
  ASR/1 -> complex_mult_w_ngtd_bi/1, Delay/1
  Register3/1 -> Q_Out/1
  Register2/1 -> I_Out/1
  complex_mult/1 -> Register/1
  complex_mult/2 -> Register1/1
  Err_Q/1 -> complex_mult/4
  Err_I/1 -> complex_mult/3
  Real-Imag to Complex1/1 -> Coeff/1
  Gateway Out1/1 -> Real-Imag to Complex1/2
  Gateway Out/1 -> Real-Imag to Complex1/1
  AddSub/1 -> sreg/1
  AddSub1/1 -> sreg1/1
  counter/1 -> ASR/2, ASR1/2
  counter/2 -> Delay1/1
  sreg/1 -> complex_mult_w_ngtd_bi/3, Gateway Out/1, AddSub/2
  Register/1 -> AddSub/1
  Register1/1 -> AddSub1/1
  Accumulator1/1 -> Register3/1
  complex_mult_w_ngtd_bi/2 -> Accumulator1/1
  complex_mult_w_ngtd_bi/1 -> Accumulator/1
  Delay1/1 -> Register3/2, Register2/2, Accumulator/2, Accumulator1/2
  Accumulator/1 -> Register2/1
  Delay/1 -> complex_mult/1
  Delay4/1 -> complex_mult/2
  sreg1/1 -> complex_mult_w_ngtd_bi/4, Gateway Out1/1, AddSub1/2
